simulink model "Simplified_Wind_Turbine_model"  (R2023b)
settings: Solver=ode23t  StartTime=0.0  StopTime=simT  RelTol=1e-3  AbsTol=1e-3
PreLoadFcn:
  | sscv_wind_turbine_input
values from neighbouring files (symbols this model uses):
  actuatorRampRate = 20    [sscv_wind_turbine_input.m]
  brakePressure = 100    [sscv_wind_turbine_input.m]
  controllerTimeConstant = 2    [sscv_wind_turbine_input.m]
  cumulativeStressThreshold = 1.5e6    (= 1500000)    [sscv_wind_turbine_input.m]
  generatorEfficiency = 90    [sscv_wind_turbine_input.m]
  iGenerationGain = 1    [sscv_wind_turbine_input.m]
  initialOperationTime = 0    [sscv_wind_turbine_input.m]
  inizialStressThreshold = 500e3    (= 500000)    [sscv_wind_turbine_input.m]
  maxPitchAngle = max(pitch)    [sscv_wind_turbine_input.m]
  minPitchAngle = min(pitch)    [sscv_wind_turbine_input.m]
  pGenerationGain = 0.1    [sscv_wind_turbine_input.m]
  pGeneratorBrakeLimit = 0.50    (= 0.5)    [sscv_wind_turbine_input.m]
  pitchBrakeAngle = 95    [sscv_wind_turbine_input.m]
  stressRateRelease = 0.05    [sscv_wind_turbine_input.m]
  transformerRatedPower = 1.8    [sscv_wind_turbine_input.m]
  turbineRatedPower = 1.5    [sscv_wind_turbine_input.m]
  vWindRated = 12    [sscv_wind_turbine_input.m]
  wAtGeneratorRatedPower = wTurbineCutOut*gearRatio    (= 1227.93)    [sscv_wind_turbine_input.m]
  wearRate = 0.033    [sscv_wind_turbine_input.m]
  wGeneratorBrakeLimit = 0.50    (= 0.5)    [sscv_wind_turbine_input.m]
  wTurbineCutOut = 22    [sscv_wind_turbine_input.m]
undefined symbols (not defined in the file or in its folder): Derating, mpptOmega, mpptPower, mpptWindSpeed
libraries: fl_lib x22, simulink x14, nesl_utility x11, sdl_lib x10, dspnetwork x3, simulink_extras x3
(part 1 of 2)
CloseFcn:
  | try,close(h_sscv_wind_turbine),end
  | clear h_sscv_wind_turbine
  | 
  | clear airDensity cp pitch TSR turbineRadius
  | clear vWindThreshold wThreshold vWindCutInLower
  | clear vWindCutOut vWindCutInUpper vWindRated
  | clear wTurbineCutIn wTurbineCutOut wTurbinePark
  | clear pitchBrakeAngle minPitchAngle maxPitchAngle
  | clear actuatorRampRate controllerTimeConstant
  | clear turbineRatedPower pGenerationGain
  | clear brakePressure brakeTorqueRadius
  | clear brakePistonArea brakeStaticFrictionCoeff
  | clear brakeKineticFrictionCoeff brakeClutchVelocityTol
  | clear brakeThresholdPressure numFrictionSurfaces
  | clear rotorBladeInertia generatorInertia
  | clear carrierShaftInertia stepShaftInertia
  | clear ringSunTeethRatio firstStepTeethRatio
  | clear secondStepTeethRatio windProfile
  | clear Derating gearRatio
  | clear generatorEfficiency mpptOmega mpptPower
  | clear generatorLumpedInductance generatorLumpedResistance
  | clear gridFrequency iGenerationGain
  | clear mpptWindSpeed transformerPrimaryVoltage
  | clear transformerRatedPower transformerSecondaryVoltage
  | clear wGeneratorBrakeLimit wAtGeneratorRatedPower
  | clear cpBraking simT pGeneratorBrakeLimit
  | clear windProfile1 windProfile2 windProfile3
  | clear numTSR
  | clear logsout_sscv_wind_turbine
  | clear simlog_sscv_wind_turbine
Description:
  | Wind Turbine
settings Model: SimulationMode=accelerator  Creator=The MathWorks, Inc.  LastModifiedBy=stefa
settings SolverCC: AutoScaleAbsTol=off  MaxConsecutiveMinStep=5  AlgebraicLoopSolver=TrustRegion  MaxZcPerStep=1
settings DataIOCC: SaveOutput=off  DSMLogging=off  SaveTime=off  ReturnWorkspaceOutputs=off  SignalLoggingName=logsout_sscv_wind_turbine
settings OptimizationCC: ReuseModelBlockBuffer=off
settings DebuggingCC: ReadBeforeWriteMsg=DisableAll  WriteAfterWriteMsg=DisableAll  WriteAfterReadMsg=DisableAll  MultiTaskDSMMsg=none  UnconnectedInputMsg=warning  UnconnectedOutputMsg=warning  UnconnectedLineMsg=warning
settings ModelReferenceCC: EnableRefExpFcnMdlSchedulingChecks=on
settings RTWCC: DLArmComputeVersion=19.05
settings SimscapeCC: SimscapeLogType=all  SimscapeLogSimulationStatistics=on  SimscapeLogName=simlog_sscv_wind_turbine  SimscapeLogDataHistory=10000000

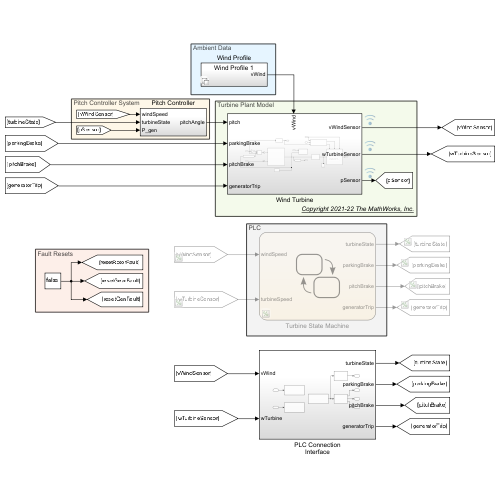
[thumbnail: Simulink's stored preview of the top-level diagram]
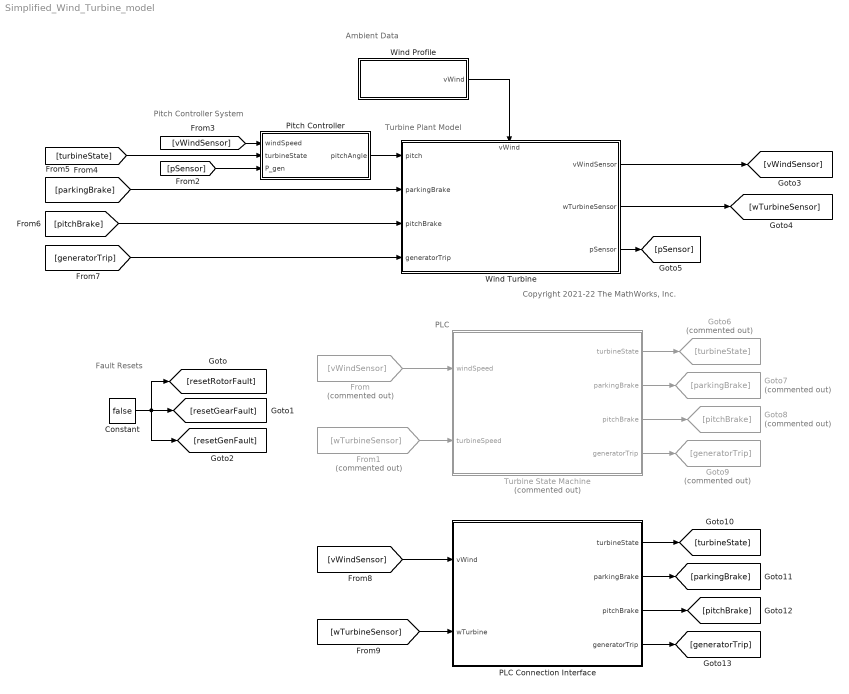
== system Simplified_Wind_Turbine_model ==
  note: Pitch Controller System
  note: Ambient Data
  note: Turbine Plant Model
  note: PLC
  note: Fault Resets
  note: Copyright 2021-22 The MathWorks, Inc.
  Constant : Constant  Value=false
  From : From  Commented=on  GotoTag=vWindSensor
  From1 : From  Commented=on  GotoTag=wTurbineSensor
  Goto6 : Goto  Commented=on  GotoTag=turbineState
  Goto7 : Goto  Commented=on  GotoTag=parkingBrake
  Goto8 : Goto  Commented=on  GotoTag=pitchBrake
  Goto9 : Goto  Commented=on  GotoTag=generatorTrip
  PLC Connection Interface : Subsystem
  Pitch Controller : Subsystem
  Turbine State Machine : Stateflow chart  Commented=on  TreatAsAtomicUnit=on
      settings: PortSchema="{\"entries\":[{\"content\":{\"sides\":[{\"content\":{\"connectorIds\":[\"In1\",\"In2\"]},\"type\":\"ConnectorPlacement.EquallySpacedRectSide\",\"uuid\":\"327e6e10-1b21-4a96-a275-8de2d485008c\"},{\"content\":{\"connectorIds\":[\"Out4\",\"Out2\",\"Out1\",\"Out3\"],\"side\":\"RIGHT\"},\"type\":\"ConnectorPlacement.EquallySpacedRectSide\",\"uuid\":\"1988adc6-59d9-4b8c-bf9e-88a31d7027f5\"},{\"content\":{\"side\":\"TOP\"},\"type\":\"ConnectorPlacement.EquallySpacedRectSide\",\"uuid\":\"79d1a7b7-1285-45ed-a7b5-26a06b144177\"}]},\"type\":\"ConnectorPlacement.EquallySpacedConnector\",\"uuid\":\"dd4ce8a9-3f97-44e2-8b7f-090ddfd1b400\"}],\"packageUris\":[\"http://schema.mathworks.com/mf0/Connector/R2020b\"],\"version\":\"1.0\"}"
  Wind Profile : Subsystem  Variant=on  VariantControl=Choice
  Wind Turbine : Subsystem
      settings: PortSchema="{\"entries\":[{\"content\":{\"sides\":[{\"content\":{\"connectorIds\":[\"In1\",\"In2\",\"In3\",\"In4\"]},\"type\":\"ConnectorPlacement.EquallySpacedRectSide\",\"uuid\":\"d7bfd4c3-1b44-42d5-b480-d0fc308ef744\"},{\"content\":{\"connectorIds\":[\"Out1\",\"Out2\",\"Out3\"],\"side\":\"RIGHT\"},\"type\":\"ConnectorPlacement.EquallySpacedRectSide\",\"uuid\":\"d62ac46e-8555-4545-8829-a8ccb57f6534\"},{\"content\":{\"connectorIds\":[\"In5\"],\"side\":\"TOP\"},\"type\":\"ConnectorPlacement.EquallySpacedRectSide\",\"uuid\":\"57f7c376-ec8e-430a-b1f8-8d8045a51355\"}]},\"type\":\"ConnectorPlacement.EquallySpacedConnector\",\"uuid\":\"f4d0f8a6-66a9-4a6a-8fc8-0ea319581c40\"}],\"packageUris\":[\"http://schema.mathworks.com/mf0/Connector/R2020b\"],\"version\":\"1.0\"}"
  wires:
  Pitch Controller/1(pitchAngle) -> Wind Turbine/1(pitch)
  Wind Profile/1(vWind) -> Wind Turbine/5(vWind)
  Constant/1 -> [resetGenFault], [resetRotorFault], [resetGearFault]
  Wind Turbine/1(vWindSensor) -> [vWindSensor]
  Wind Turbine/2(wTurbineSensor) -> [wTurbineSensor]
  Wind Turbine/3(pSensor) -> [pSensor]
  From/1 -> Turbine State Machine/1(windSpeed)
  From1/1 -> Turbine State Machine/2(turbineSpeed)
  [pSensor] -> Pitch Controller/3(P_gen)
  [vWindSensor] -> Pitch Controller/1(windSpeed)
  Turbine State Machine/4(turbineState) -> Goto6/1
  Turbine State Machine/2(parkingBrake) -> Goto7/1
  Turbine State Machine/1(pitchBrake) -> Goto8/1
  Turbine State Machine/3(generatorTrip) -> Goto9/1
  [turbineState] -> Pitch Controller/2(turbineState)
  [parkingBrake] -> Wind Turbine/2(parkingBrake)
  [pitchBrake] -> Wind Turbine/3(pitchBrake)
  [generatorTrip] -> Wind Turbine/4(generatorTrip)
  [vWindSensor] -> PLC Connection Interface/1(vWind)
  [wTurbineSensor] -> PLC Connection Interface/2(wTurbine)
  PLC Connection Interface/2(parkingBrake) -> [parkingBrake]
  PLC Connection Interface/1(turbineState) -> [turbineState]
  PLC Connection Interface/3(pitchBrake) -> [pitchBrake]
  PLC Connection Interface/4(generatorTrip) -> [generatorTrip]

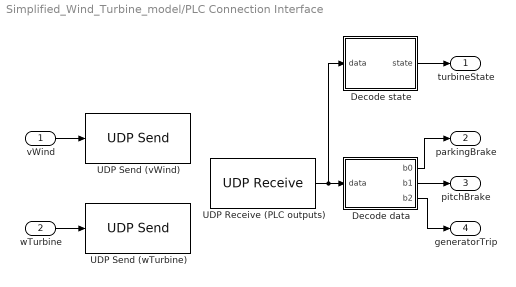
== system Simplified_Wind_Turbine_model/PLC Connection Interface ==
  vWind : Inport
  wTurbine : Inport  Port=2
  Decode data : MATLAB Function  TreatAsAtomicUnit=on
  Decode state : MATLAB Function  TreatAsAtomicUnit=on
  UDP Receive (PLC outputs) : dspnetwork/UDP Receive  localURL='0.0.0.0'  localPort=25000  remoteURL='0.0.0.0'  remotePort=-1  recvBufferSize=8192  dims=255  signalDatatype=uint8  isComplex=off  isVarSize=on  showBlockingTime=off  blockingTime=0  sampletime=0.1  blockPlatform=[]
      settings: LibrarySourceBlock=dspsrcs4/UDP Receive
  UDP Send (vWind) : dspnetwork/UDP Send  remoteURL='127.0.0.1'  remotePort=25000  localURL='0.0.0.0'  localPortSource=Automatically determine  localPort=-1  sendBufferSize=8192  sampletime=-1  blockPlatform=[]  separateLengthPort=0
      settings: LibrarySourceBlock=dspsnks4/UDP Send
  UDP Send (wTurbine) : dspnetwork/UDP Send  remoteURL='127.0.0.1'  remotePort=25000  localURL='0.0.0.0'  localPortSource=Automatically determine  localPort=-1  sendBufferSize=8192  sampletime=-1  blockPlatform=[]  separateLengthPort=0
      settings: LibrarySourceBlock=dspsnks4/UDP Send
  turbineState : Outport
  parkingBrake : Outport  Port=2
  pitchBrake : Outport  Port=3
  generatorTrip : Outport  Port=4
  wires:
  UDP Receive (PLC outputs)/1 -> Decode state/1(data), Decode data/1(data)
  Decode data/1(b0) -> parkingBrake/1
  Decode data/2(b1) -> pitchBrake/1
  Decode data/3(b2) -> generatorTrip/1
  Decode state/1(state) -> turbineState/1
  vWind/1 -> UDP Send (vWind)/1
  wTurbine/1 -> UDP Send (wTurbine)/1

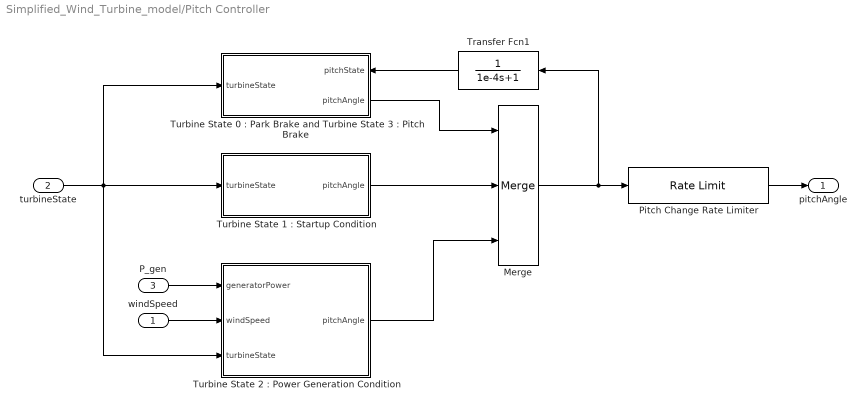
== system Simplified_Wind_Turbine_model/Pitch Controller ==
  windSpeed : Inport
  turbineState : Inport  Port=2
  P_gen : Inport  Port=3
  Merge : Merge  Inputs=3
  Pitch Change Rate Limiter : RateLimiter  RisingSlewLimit=actuatorRampRate  FallingSlewLimit=-actuatorRampRate  SampleTimeMode=inherited
  Transfer Fcn1 : TransferFcn  Denominator=[1e-4 1]
  "Turbine State 0 : Park Brake and Turbine State 3 : Pitch Brake" : Subsystem
      settings: PortSchema="{\"entries\":[{\"content\":{\"sides\":[{\"content\":{\"connectorIds\":[\"In1\"]},\"type\":\"ConnectorPlacement.EquallySpacedRectSide\",\"uuid\":\"c81c0fc4-0b31-4a43-acf3-ef02f67f12ef\"},{\"content\":{\"connectorIds\":[\"In2\",\"Out1\"],\"side\":\"RIGHT\"},\"type\":\"ConnectorPlacement.EquallySpacedRectSide\",\"uuid\":\"c20c9bc8-a4c7-4c6f-a8fa-fe8ff88298f7\"},{\"content\":{\"connectorIds\":[],\"side\":\"TOP\"},\"type\":\"ConnectorPlacement.EquallySpacedRectSide\",\"uuid\":\"2b845051-401f-423c-a453-0a1243a015d1\"}]},\"type\":\"ConnectorPlacement.EquallySpacedConnector\",\"uuid\":\"502647d6-ee95-4637-92b5-6d3c38784edf\"}],\"packageUris\":[\"http://schema.mathworks.com/mf0/Connector/R2020b\"],\"version\":\"1.0\"}"
  "Turbine State 1 : Startup Condition" : Subsystem
  "Turbine State 2 : Power Generation Condition" : Subsystem
  pitchAngle : Outport
  wires:
  Pitch Change Rate Limiter/1 -> pitchAngle/1
  turbineState/1 -> "Turbine State 2 : Power Generation Condition"/3(turbineState), "Turbine State 0 : Park Brake and Turbine State 3 : Pitch Brake"/1(turbineState), "Turbine State 1 : Startup Condition"/1(turbineState)
  P_gen/1 -> "Turbine State 2 : Power Generation Condition"/1(generatorPower)
  Merge/1 -> Pitch Change Rate Limiter/1, Transfer Fcn1/1
  "Turbine State 0 : Park Brake and Turbine State 3 : Pitch Brake"/1(pitchAngle) -> Merge/1
  "Turbine State 1 : Startup Condition"/1(pitchAngle) -> Merge/2
  "Turbine State 2 : Power Generation Condition"/1(pitchAngle) -> Merge/3
  windSpeed/1 -> "Turbine State 2 : Power Generation Condition"/2(windSpeed)
  Transfer Fcn1/1 -> "Turbine State 0 : Park Brake and Turbine State 3 : Pitch Brake"/2(pitchState)

== system Simplified_Wind_Turbine_model/Wind Profile ==
  Wind Profile 1 : Subsystem  VariantControl=windProfile1
  Wind Profile 2 : Subsystem  VariantControl=windProfile2
  Wind Profile 3 : Subsystem  VariantControl=windProfile3
  vWind : Outport

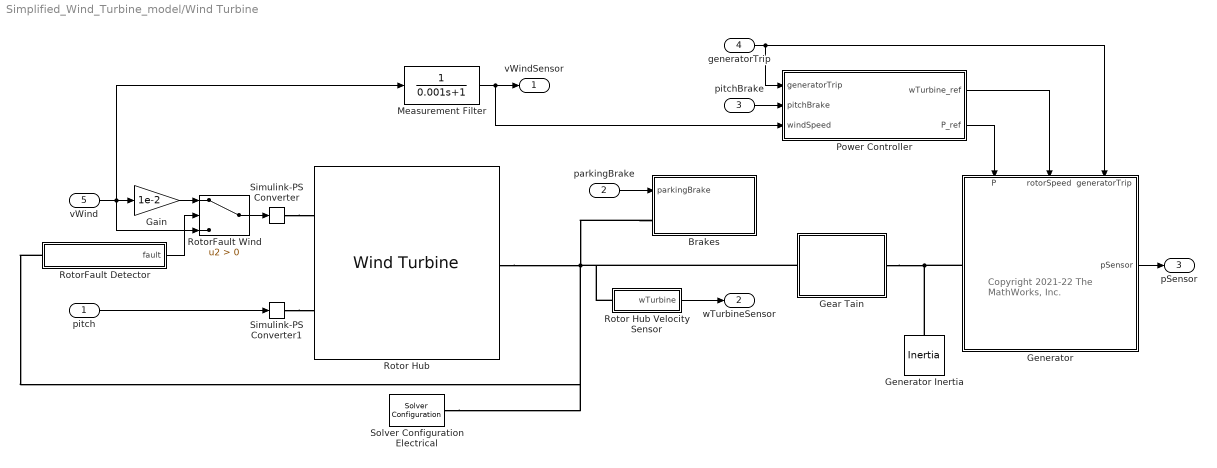
== system Simplified_Wind_Turbine_model/Wind Turbine ==
  note: Copyright 2021-22
      | The MathWorks, Inc.
  pitch : Inport
  parkingBrake : Inport  Port=2
  pitchBrake : Inport  Port=3
  generatorTrip : Inport  Port=4
  vWind : Inport  Port=5
  Brakes : Subsystem
  Gain : Gain  Gain=1e-2
  Gear Tain : Subsystem
  Generator : Subsystem
      settings: PortSchema="{\"entries\":[{\"content\":{\"sides\":[{\"content\":{\"connectorIds\":[\"LConn1\"]},\"type\":\"ConnectorPlacement.EquallySpacedRectSide\",\"uuid\":\"7b4c28dc-15ef-4b85-b689-03d2480b533c\"},{\"content\":{\"connectorIds\":[\"Out1\"],\"side\":\"RIGHT\"},\"type\":\"ConnectorPlacement.EquallySpacedRectSide\",\"uuid\":\"eb8f45a7-b1c6-4508-84d0-11c24daa06af\"},{\"content\":{\"connectorIds\":[\"In1\",\"In2\",\"In3\"],\"side\":\"TOP\"},\"type\":\"ConnectorPlacement.EquallySpacedRectSide\",\"uuid\":\"25f559ac-6538-4a67-925f-810721e5a71b\"},{\"content\":{\"side\":\"BOTTOM\"},\"type\":\"ConnectorPlacement.EquallySpacedRectSide\",\"uuid\":\"5619365a-5656-4cf0-a126-06e5a3f6ebac\"}]},\"type\":\"ConnectorPlacement.EquallySpacedConnector\",\"uuid\":\"4c1773ae-12cd-4fd2-b48a-ee13558bc69b\"}],\"packageUris\":[\"http://schema.mathworks.com/mf0/Connector/R2020b\"],\"version\":\"1.0\"}"
  Generator Inertia : fl_lib/Mechanical/Rotational Elements/Inertia  inertia=generatorInertia kg*m^2  num_ports=foundation.enum.numPorts2.one  w_specify=on  w_priority=None  w=0 rad/s  w_nominal_specify=off  w_nominal_unit=rad/s  w_nominal_value=1  t_specify=off  t_priority=None  t=0 N*m  t_nominal_specify=off  t_nominal_unit=N*m  t_nominal_value=1
  Measurement Filter : TransferFcn  Denominator=[0.001 1]
  Power Controller : Subsystem
  Rotor Hub : sdl_lib/Engines & Motors/Wind Turbine  model_thrust=false  R_rotor=turbineRadius m  pitch_TLU=pitch deg  lambda_TLU=TSR  Cp_TLU=cp  Ct_TLU=[0.0777, 0.1421, 0.3753, 0.6599, 0.8160, 0.9112, 0.9925, 1.0708, 1.1147; 0.0762, 0.1377, 0.3570, 0.5529, 0.6291, 0.6573, 0.6706, 0.6421, 0.6284; 0.0682, 0.1292, 0.3362, 0.4664, 0.4874, 0.4547, 0.3915, 0.2865, 0.2249; -0.05 * ones(1, 9)]  rho_air=airDensity kg/m^3  model_inertia=sdl.enum.model_inertia.on  rotor_inertia=rotorBladeInertia kg*m^2  init_rot_vel=0 rad/s  v_thr=0.01 m/s  w_thr=0.01 rad/s  expose_port_C=0
      settings: InternalSimscapePortConfiguration="{\"Bottom\":[],\"Left\":[{\"id\":\"vWind\",\"label\":\"V\",\"type\":\"input\"},{\"id\":\"pitch\",\"label\":\"β\",\"type\":\"input\"}],\"Right\":[{\"id\":\"R\",\"label\":\"R\",\"type\":\"foundation.mechanical.rotational.rotational\"}],\"Top\":[]}"
  Rotor Hub Velocity Sensor : Subsystem
  RotorFault Detector : Subsystem
  RotorFault Wind : Switch  Criteria=u2 > Threshold  SaturateOnIntegerOverflow=off  InputSameDT=off
  Simulink-PS Converter : nesl_utility/Simulink-PS Converter  PhysicalDomain=network_engine_domain  SubClassName=ps_input  LeftPortType=input  RightPortType=output  PseudoPeriodic=off  Frequencies=[]  NoiseDistribution=none  NoiseParameters=[]  Unit=m/s  AffineConversion=off  FilteringAndDerivatives=filter  SimscapeFilterOrder=1  InputFilterTimeConstant=0.001  UdotUserProvided=0
  Simulink-PS Converter1 : nesl_utility/Simulink-PS Converter  PhysicalDomain=network_engine_domain  SubClassName=ps_input  LeftPortType=input  RightPortType=output  PseudoPeriodic=off  Frequencies=[]  NoiseDistribution=none  NoiseParameters=[]  Unit=deg  AffineConversion=off  FilteringAndDerivatives=filter  SimscapeFilterOrder=1  InputFilterTimeConstant=0.001  UdotUserProvided=0
  Solver Configuration Electrical : nesl_utility/Solver Configuration  PhysicalDomain=network_engine_domain  SubClassName=solver  LeftPortType=input  RightPortType=generic  Tones=[]  Harmonics=[]  SimulateNoise=off  Profile=off  UseLocalSampling=off  EnableSwitchedLinearOptims=on  FrequencyDomain=off  UseCCode=off  RelTol=0.001  AbsTol=0.001  MinStep=1e-09  ToWorkspace=off  RevertToSquareIcSolve=off  NumHomotopyIterations=100  PhasorMode=off  PhasorModeNumHarmonics=1  ConsistencySolver=NEWTON_FTOL  IndexReductionMethod=DerivativeReplacement  DoDC=off  ResidualTolerance=1e-09  ConsistencyTolSource=GLOBAL  ConsistencyAbsTol=0.001  ConsistencyRelTol=0.001  ConsistencyTolFactor=0.001  UseLocalSolver=off  LocalSolverChoice=NE_TRAPEZOIDAL_ADVANCER  ResolveIndetEquations=on  FunctionEvalNumThread=1  LocalSolverSampleTime=1e-5  DoFixedCost=off  MaxNonlinIter=3  MaxModeIter=2  ComputeImpulses=off  ImpulseIterations=2  LinearAlgebra=auto  LinearAlgebraNumThread=0  EquationFormulation=NE_TIME_EF  DelaysMemoryBudget=1024  AutomaticFiltering=on  FilteringTimeConstant=0.001  PartitionStorageMethod=AS_NEEDED  PartitionMemoryBudget=1024  PartitionMethod=ROBUST  MultibodyUseLocalSolver=off  MultibodyLocalSolverChoice=ODE1  MultibodyLocalSolverSampleTime=0.001
  vWindSensor : Outport
  wTurbineSensor : Outport  Port=2
  pSensor : Outport  Port=3
  wires:
  Rotor Hub Velocity Sensor/1(wTurbine) -> wTurbineSensor/1
  Power Controller/2(P_ref) -> Generator/1(P)
  Generator/1(pSensor) -> pSensor/1
  parkingBrake/1 -> Brakes/1(parkingBrake)
  generatorTrip/1 -> Power Controller/1(generatorTrip), Generator/3(generatorTrip)
  Measurement Filter/1 -> vWindSensor/1, Power Controller/3(windSpeed)
  Power Controller/1(wTurbine_ref) -> Generator/2(rotorSpeed)
  pitchBrake/1 -> Power Controller/2(pitchBrake)
  pitch/1 -> Simulink-PS Converter1/1
  vWind/1 -> Measurement Filter/1, RotorFault Wind/3, Gain/1
  RotorFault Wind/1 -> Simulink-PS Converter/1
  RotorFault Detector/1(fault) -> RotorFault Wind/2
  Gain/1 -> RotorFault Wind/1
  connections:
  Generator/LConn1 -- Gear Tain/RConn1 -- Generator Inertia/LConn1
  Rotor Hub/RConn1 -- Solver Configuration Electrical/RConn1 -- RotorFault Detector/LConn1 -- Rotor Hub Velocity Sensor/LConn1 -- Gear Tain/LConn1 -- Brakes/LConn1
  Simulink-PS Converter/RConn1 -- Rotor Hub/LConn1
  Simulink-PS Converter1/RConn1 -- Rotor Hub/LConn2

== system Simplified_Wind_Turbine_model/Pitch Controller/Turbine State 0 : Park Brake and Turbine State 3 : Pitch Brake ==
  turbineState : Inport
  pitchState : Inport  Port=2
  Compare To Constant : simulink/Logic and Bit Operations/Compare To Constant  relop===  const=0  OutDataTypeStr=boolean
  Compare To Constant1 : simulink/Logic and Bit Operations/Compare To Constant  relop===  const=3  OutDataTypeStr=boolean
  OR : Logic  Operator=OR  IconShape=distinctive  AllPortsSameDT=off  OutDataTypeStr=boolean
  Turbine State 0 an 3 : Subsystem
  pitchAngle : Outport
  wires:
  Turbine State 0 an 3/1(pitchAngle) -> pitchAngle/1
  turbineState/1 -> Compare To Constant1/1, Compare To Constant/1
  pitchState/1 -> Turbine State 0 an 3/1(pitchState)
  OR/1 -> Turbine State 0 an 3/Enable
  Compare To Constant/1 -> OR/1
  Compare To Constant1/1 -> OR/2

== system Simplified_Wind_Turbine_model/Pitch Controller/Turbine State 1 : Startup Condition ==
  turbineState : Inport
  Compare To Constant : simulink/Logic and Bit Operations/Compare To Constant  relop===  const=1  OutDataTypeStr=boolean
  Turbine State 1 : Subsystem
  pitchAngle : Outport
  wires:
  turbineState/1 -> Compare To Constant/1
  Compare To Constant/1 -> Turbine State 1/Enable
  Turbine State 1/1(pitchAngle) -> pitchAngle/1

== system Simplified_Wind_Turbine_model/Pitch Controller/Turbine State 2 : Power Generation Condition ==
  generatorPower : Inport
  windSpeed : Inport  Port=2
  turbineState : Inport  Port=3
  Compare To Constant : simulink/Logic and Bit Operations/Compare To Constant  relop===  const=2  OutDataTypeStr=boolean
  Turbine State 2 : Subsystem
  pitchAngle : Outport
  wires:
  Turbine State 2/1(pitchAngle) -> pitchAngle/1
  Compare To Constant/1 -> Turbine State 2/Enable
  turbineState/1 -> Compare To Constant/1
  generatorPower/1 -> Turbine State 2/1(generatorPower)
  windSpeed/1 -> Turbine State 2/2(windSpeed)

== system Simplified_Wind_Turbine_model/Wind Profile/Wind Profile 1 ==
  Ramp : simulink/Sources/Ramp  slope=1  start=45  InitialOutput=15
  Saturation : Saturate  UpperLimit=22  LowerLimit=0
  vWind : Outport
  wires:
  Ramp/1 -> Saturation/1
  Saturation/1 -> vWind/1

== system Simplified_Wind_Turbine_model/Wind Profile/Wind Profile 2 ==
  Add : Sum  Inputs=+
  Mux : Mux  Inputs=3
  Ramp : simulink/Sources/Ramp  slope=0.7  start=0  InitialOutput=0
  Ramp1 : simulink/Sources/Ramp  slope=0.7  start=115  InitialOutput=0
  Ramp2 : simulink/Sources/Ramp  slope=-0.7  start=160  InitialOutput=0
  Saturation : Saturate  UpperLimit=10  LowerLimit=0
  Saturation1 : Saturate  UpperLimit=12  LowerLimit=0
  Saturation2 : Saturate  UpperLimit=0  LowerLimit=-7
  vWind : Outport
  wires:
  Saturation1/1 -> Mux/2
  Ramp/1 -> Saturation/1
  Ramp2/1 -> Saturation2/1
  Add/1 -> vWind/1
  Saturation/1 -> Mux/1
  Ramp1/1 -> Saturation1/1
  Mux/1 -> Add/1
  Saturation2/1 -> Mux/3

== system Simplified_Wind_Turbine_model/Wind Profile/Wind Profile 3 ==
  Ramp : simulink/Sources/Ramp  slope=1  start=45  InitialOutput=15
  Saturation : Saturate  UpperLimit=17  LowerLimit=0
  vWind : Outport
  wires:
  Ramp/1 -> Saturation/1
  Saturation/1 -> vWind/1

== system Simplified_Wind_Turbine_model/Wind Turbine/Brakes ==
  parkingBrake : Inport
  Disk Friction Clutch : sdl_lib/Clutches/Disc Friction Clutch  geometry_model=1  r_eff=brakeTorqueRadius m  d_o=150 mm  d_i=100 mm  nS=numFrictionSurfaces  piston_area=brakePistonArea m^2  unidirectional=0  friction_model=1  mu_w_vector=[1 1e8] rad/s  temperature_TLU=[280.0, 300.0, 320.0] K  mu_static=brakeStaticFrictionCoeff  mu_static_vector=[0.4, 0.38, 0.36]  mu_coulomb=brakeKineticFrictionCoeff  mu_coulomb_vector=[0.3 0.001]  mu_coulomb_temp_vector=[0.3, 0.28, 0.25]  mu_coulomb_matrix=[0.34, 0.32, 0.3; 0.3, 0.28, 0.25; 0.25, 0.2, 0.15]  mu_interp_method=1  mu_extrap_method=1  d_f=1  w_tol=brakeClutchVelocityTol rad/s  pressure_min=brakeThresholdPressure Pa  mu_visc=0 N*m/(rad/s)  initial_state_locked=sdl.enum.initial_lock.unlocked  enable_faults=simscape.enum.onoff.off  fault_type=sdl.enum.clutchFault.lock  external_fault=simscape.enum.onoff.off  temporal_fault=simscape.enum.onoff.off  fault_time=5 s  report_fault=simscape.enum.assert.action.none  thermal_mass=25 kJ/K  T_init=300 K
      settings: InternalSimscapePortConfiguration="{\"Bottom\":[],\"Left\":[{\"id\":\"P\",\"label\":\"P\",\"type\":\"input\"},{\"id\":\"B\",\"label\":\"B\",\"type\":\"foundation.mechanical.rotational.rotational\"}],\"Right\":[{\"id\":\"F\",\"label\":\"F\",\"type\":\"foundation.mechanical.rotational.rotational\"}],\"Top\":[]}"
  Engagement Pressure : Gain  Gain=brakePressure
  Mechanical Rotational Reference : fl_lib/Mechanical/Rotational Elements/Mechanical Rotational Reference
  Simulink-PS Converter : nesl_utility/Simulink-PS Converter  PhysicalDomain=network_engine_domain  SubClassName=ps_input  LeftPortType=input  RightPortType=output  PseudoPeriodic=off  Frequencies=[]  NoiseDistribution=none  NoiseParameters=[]  Unit=bar  AffineConversion=off  FilteringAndDerivatives=zero  SimscapeFilterOrder=1  InputFilterTimeConstant=0.005  UdotUserProvided=0
  R : PMIOPort  Tag=PMCPort  Side=Left
  wires:
  Engagement Pressure/1 -> Simulink-PS Converter/1
  parkingBrake/1 -> Engagement Pressure/1
  connections:
  Disk Friction Clutch/RConn1 -- Mechanical Rotational Reference/LConn1
  R/RConn1 -- Disk Friction Clutch/LConn2
  Simulink-PS Converter/RConn1 -- Disk Friction Clutch/LConn1

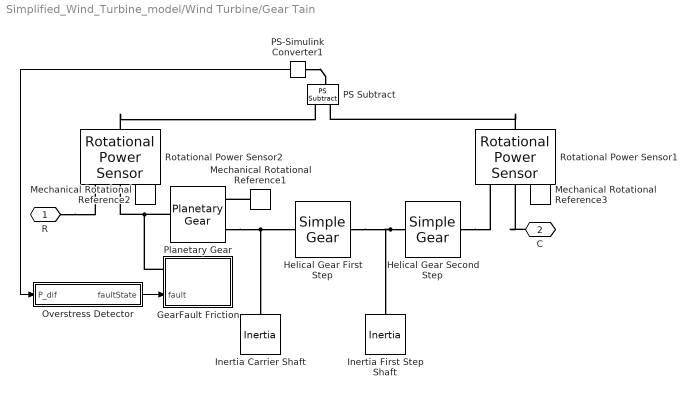
== system Simplified_Wind_Turbine_model/Wind Turbine/Gear Tain ==
  GearFault Friction : Subsystem
      settings: PortSchema="{\"entries\":[{\"content\":{\"sides\":[{\"content\":{\"connectorIds\":[\"LConn1\",\"In1\"]},\"type\":\"ConnectorPlacement.EquallySpacedRectSide\",\"uuid\":\"22e76782-3382-417d-ae5a-a7b1043ec7fc\"},{\"content\":{\"side\":\"RIGHT\"},\"type\":\"ConnectorPlacement.EquallySpacedRectSide\",\"uuid\":\"493f48a2-9880-444c-a7eb-314aeba6f102\"},{\"content\":{\"side\":\"TOP\"},\"type\":\"ConnectorPlacement.EquallySpacedRectSide\",\"uuid\":\"41df36c8-e029-4ee0-982b-378728ae749a\"}]},\"type\":\"ConnectorPlacement.EquallySpacedConnector\",\"uuid\":\"9c211b33-7010-4c0e-a899-cbcb07dff7a9\"}],\"packageUris\":[\"http://schema.mathworks.com/mf0/Connector/R2020b\"],\"version\":\"1.0\"}"
  Helical Gear First Step : sdl_lib/Gears/Simple Gear  ratio=firstStepTeethRatio  rotation_direction=sdl.enum.shaftOutputDirection.opposite  friction_model=sdl.enum.gear_efficiencies_load.constant  T_noload=0.1 N*m  T_nom=5 N*m  efficiency_nom=0.8  efficiency=0.95  temperature_TLU=[ 280 300 320 ] K  load_TLU=[ 1 5 10 ] N*m  efficiency_TLU=[ 0.95 0.9 0.85 ]  efficiency_TLU2=[ 0.85 0.8 0.75; 0.95 0.9 0.85; 0.85 0.8 0.7 ]  w_thr=0.01 rad/s  pwr_thr=0.001 W  enable_backlash=false  hardstop_model=simscape.enum.hardstop.smooth  backlash_distance=1e-3 mm  r_base=0.1 m  transition=1e-4 mm  backlash_stiffness=1e7 N/m  backlash_damping=1e6 N/(m/s)  coeff_rest=0  v_tol=0.001 m/s  f_tol=0 N  mu_visc=[ 0 0 ] N*m/(rad/s)  enable_faults=simscape.enum.onoff.off  efficiency_fault=0.05  external_fault=simscape.enum.onoff.off  temporal_fault=simscape.enum.onoff.off  fault_time=5 s  fault_angles=pi / 12 rad  report_fault=simscape.enum.assert.action.none  thermal_mass=50 J/K  temperature_specify=off  temperature_priority=High  temperature=300 K  temperature_nominal_specify=off  temperature_nominal_unit=K  temperature_nominal_value=1  x_backlash_specify=off  x_backlash_priority=None  x_backlash=0 mm  x_backlash_nominal_specify=off  x_backlash_nominal_unit=mm  x_backlash_nominal_value=1  f_hardstop_specify=off  f_hardstop_priority=None  f_hardstop=0 N  f_hardstop_nominal_specify=off  f_hardstop_nominal_unit=N  f_hardstop_nominal_value=1  v_backlash_specify=off  v_backlash_priority=None  v_backlash=0 m/s  v_backlash_nominal_specify=off  v_backlash_nominal_unit=m/s  v_backlash_nominal_value=1
  Helical Gear Second Step : sdl_lib/Gears/Simple Gear  ratio=secondStepTeethRatio  rotation_direction=sdl.enum.shaftOutputDirection.same  friction_model=sdl.enum.gear_efficiencies_load.constant  T_noload=0.1 N*m  T_nom=5 N*m  efficiency_nom=0.8  efficiency=0.95  temperature_TLU=[ 280 300 320 ] K  load_TLU=[ 1 5 10 ] N*m  efficiency_TLU=[ 0.95 0.9 0.85 ]  efficiency_TLU2=[ 0.85 0.8 0.75; 0.95 0.9 0.85; 0.85 0.8 0.7 ]  w_thr=0.01 rad/s  pwr_thr=0.001 W  enable_backlash=false  hardstop_model=simscape.enum.hardstop.smooth  backlash_distance=1e-3 mm  r_base=0.1 m  transition=1e-4 mm  backlash_stiffness=1e7 N/m  backlash_damping=1e6 N/(m/s)  coeff_rest=0  v_tol=0.001 m/s  f_tol=0 N  mu_visc=[ 0 0 ] N*m/(rad/s)  enable_faults=simscape.enum.onoff.off  efficiency_fault=0.05  external_fault=simscape.enum.onoff.off  temporal_fault=simscape.enum.onoff.off  fault_time=5 s  fault_angles=pi / 12 rad  report_fault=simscape.enum.assert.action.none  thermal_mass=50 J/K  temperature_specify=off  temperature_priority=High  temperature=300 K  temperature_nominal_specify=off  temperature_nominal_unit=K  temperature_nominal_value=1  x_backlash_specify=off  x_backlash_priority=None  x_backlash=0 mm  x_backlash_nominal_specify=off  x_backlash_nominal_unit=mm  x_backlash_nominal_value=1  f_hardstop_specify=off  f_hardstop_priority=None  f_hardstop=0 N  f_hardstop_nominal_specify=off  f_hardstop_nominal_unit=N  f_hardstop_nominal_value=1  v_backlash_specify=off  v_backlash_priority=None  v_backlash=0 m/s  v_backlash_nominal_specify=off  v_backlash_nominal_unit=m/s  v_backlash_nominal_value=1
  Inertia Carrier Shaft : fl_lib/Mechanical/Rotational Elements/Inertia  inertia=carrierShaftInertia kg*m^2  num_ports=foundation.enum.numPorts2.one  w_specify=on  w_priority=None  w=0 rad/s  w_nominal_specify=off  w_nominal_unit=rad/s  w_nominal_value=1  t_specify=off  t_priority=High  t=0 N*m  t_nominal_specify=off  t_nominal_unit=N*m  t_nominal_value=1
  Inertia First Step Shaft : fl_lib/Mechanical/Rotational Elements/Inertia  inertia=stepShaftInertia kg*m^2  num_ports=foundation.enum.numPorts2.one  w_specify=on  w_priority=None  w=0 rad/s  w_nominal_specify=off  w_nominal_unit=rad/s  w_nominal_value=1  t_specify=off  t_priority=High  t=0 N*m  t_nominal_specify=off  t_nominal_unit=N*m  t_nominal_value=1
  Mechanical Rotational Reference1 : fl_lib/Mechanical/Rotational Elements/Mechanical Rotational Reference
  Mechanical Rotational Reference2 : fl_lib/Mechanical/Rotational Elements/Mechanical Rotational Reference
  Mechanical Rotational Reference3 : fl_lib/Mechanical/Rotational Elements/Mechanical Rotational Reference
  Overstress Detector : Subsystem
  PS Subtract : fl_lib/Physical Signals/Functions/PS Subtract
  PS-Simulink Converter1 : nesl_utility/PS-Simulink Converter  PhysicalDomain=network_engine_domain  SubClassName=ps_output  LeftPortType=input  RightPortType=output  PseudoPeriodic=off  Frequencies=[]  VectorFormat=inherit  Unit=inherit  AffineConversion=off
  Planetary Gear : sdl_lib/Gears/Planetary Gear  rs_ratio=ringSunTeethRatio  friction_model=sdl.enum.gear_friction.constant  efficiency=[ 0.95 0.95 ]  temperature_TLU=[ 280 300 320 ] K  efficiency_sp_TLU=[ 0.95 0.9 0.85 ]  efficiency_rp_TLU=[ 0.95 0.9 0.85 ]  pwr_thr=[ 0.001 0.001 ] W  mu_visc=[0 0] N*m/(rad/s)  model_inertia=simscape.enum.onoff.off  planet_inertia=0.001 kg*m^2  thermal_mass=50 J/K  T_init=300 K
  Rotational Power Sensor1 : sdl_lib/Sensors/Rotational Power Sensor  measurement_type=sdl.enum.rotationalPowerSensorType.instantaneous  averaging_period=1 s  max_frequency=1000 Hz  max_speed=1000 rpm
      settings: InternalSimscapePortConfiguration="{\"Bottom\":[],\"Left\":[{\"id\":\"S\",\"label\":\"S\",\"type\":\"foundation.mechanical.rotational.rotational\"},{\"id\":\"R\",\"label\":\"R\",\"type\":\"foundation.mechanical.rotational.rotational\"},{\"id\":\"C\",\"label\":\"C\",\"type\":\"foundation.mechanical.rotational.rotational\"}],\"Right\":[{\"id\":\"P\",\"label\":\"P\",\"type\":\"output\"}],\"Top\":[]}"
  Rotational Power Sensor2 : sdl_lib/Sensors/Rotational Power Sensor  measurement_type=sdl.enum.rotationalPowerSensorType.instantaneous  averaging_period=1 s  max_frequency=1000 Hz  max_speed=1000 rpm
      settings: InternalSimscapePortConfiguration="{\"Bottom\":[],\"Left\":[{\"id\":\"S\",\"label\":\"S\",\"type\":\"foundation.mechanical.rotational.rotational\"},{\"id\":\"R\",\"label\":\"R\",\"type\":\"foundation.mechanical.rotational.rotational\"},{\"id\":\"C\",\"label\":\"C\",\"type\":\"foundation.mechanical.rotational.rotational\"}],\"Right\":[{\"id\":\"P\",\"label\":\"P\",\"type\":\"output\"}],\"Top\":[]}"
  R : PMIOPort  Side=Left
  C : PMIOPort  Port=2  Side=Right
  wires:
  Overstress Detector/1(faultState) -> GearFault Friction/1(fault)
  PS-Simulink Converter1/1 -> Overstress Detector/1(P_dif)
  connections:
  Planetary Gear/RConn2 -- Inertia Carrier Shaft/LConn1 -- Helical Gear First Step/RConn1
  Helical Gear Second Step/RConn1 -- Inertia First Step Shaft/LConn1 -- Helical Gear First Step/LConn1
  Mechanical Rotational Reference1/LConn1 -- Planetary Gear/RConn1
  Helical Gear Second Step/LConn1 -- Rotational Power Sensor1/LConn1
  C/RConn1 -- Rotational Power Sensor1/LConn2
  Mechanical Rotational Reference3/LConn1 -- Rotational Power Sensor1/LConn3
  Mechanical Rotational Reference2/LConn1 -- Rotational Power Sensor2/LConn3
  Planetary Gear/LConn1 -- GearFault Friction/LConn1 -- Rotational Power Sensor2/LConn2
  R/RConn1 -- Rotational Power Sensor2/LConn1
  Rotational Power Sensor1/RConn1 -- PS Subtract/LConn2
  PS-Simulink Converter1/LConn1 -- PS Subtract/RConn1
  Rotational Power Sensor2/RConn1 -- PS Subtract/LConn1

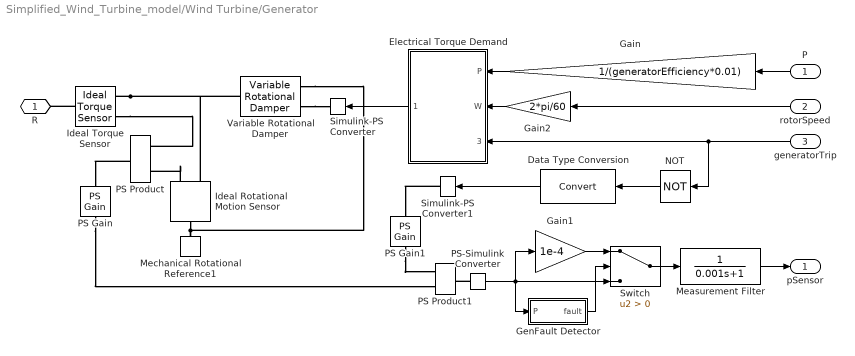
== system Simplified_Wind_Turbine_model/Wind Turbine/Generator ==
  P : Inport
  rotorSpeed : Inport  Port=2
  generatorTrip : Inport  Port=3
  Data Type Conversion : DataTypeConversion  SaturateOnIntegerOverflow=off  RndMeth=Floor
  Electrical Torque Demand : Subsystem
  Gain : Gain  Gain=1/(generatorEfficiency*0.01)
  Gain1 : Gain  Gain=1e-4
  Gain2 : Gain  Gain=2*pi/60
  GenFault Detector : Subsystem
  Ideal Rotational Motion Sensor : fl_lib/Mechanical/Mechanical Sensors/Ideal Rotational Motion Sensor  reference=foundation.enum.MeasurementReference.difference  acceleration_port=false  velocity_port=true  position_port=false  wrap_angle=simscape.enum.onoff.off  offset=0 rad
      settings: InternalSimscapePortConfiguration="{\"Bottom\":[],\"Left\":[{\"id\":\"R\",\"label\":\"R\",\"type\":\"foundation.mechanical.rotational.rotational\"}],\"Right\":[{\"id\":\"C\",\"label\":\"C\",\"type\":\"foundation.mechanical.rotational.rotational\"},{\"id\":\"W\",\"label\":\"W\",\"type\":\"output\"}],\"Top\":[]}"
  Ideal Torque Sensor : fl_lib/Mechanical/Mechanical Sensors/Ideal Torque Sensor
  Measurement Filter : TransferFcn  Denominator=[0.001 1]
  Mechanical Rotational Reference1 : fl_lib/Mechanical/Rotational Elements/Mechanical Rotational Reference
  NOT : Logic  Operator=NOT  IconShape=distinctive  AllPortsSameDT=off  OutDataTypeStr=boolean
  PS Gain : fl_lib/Physical Signals/Functions/PS Gain  gain=generatorEfficiency*0.01
  PS Gain1 : fl_lib/Physical Signals/Functions/PS Gain  gain=-1
  PS Product : fl_lib/Physical Signals/Functions/PS Product
  PS Product1 : fl_lib/Physical Signals/Functions/PS Product
  PS-Simulink Converter : nesl_utility/PS-Simulink Converter  PhysicalDomain=network_engine_domain  SubClassName=ps_output  LeftPortType=input  RightPortType=output  PseudoPeriodic=off  Frequencies=[]  VectorFormat=inherit  Unit=MW  AffineConversion=off
  Simulink-PS Converter : nesl_utility/Simulink-PS Converter  PhysicalDomain=network_engine_domain  SubClassName=ps_input  LeftPortType=input  RightPortType=output  PseudoPeriodic=off  Frequencies=[]  NoiseDistribution=none  NoiseParameters=[]  Unit=N*m/(rad/s)  AffineConversion=off  FilteringAndDerivatives=provide  SimscapeFilterOrder=1  InputFilterTimeConstant=0.001  UdotUserProvided=0
  Simulink-PS Converter1 : nesl_utility/Simulink-PS Converter  PhysicalDomain=network_engine_domain  SubClassName=ps_input  LeftPortType=input  RightPortType=output  PseudoPeriodic=off  Frequencies=[]  NoiseDistribution=none  NoiseParameters=[]  Unit=1  AffineConversion=off  FilteringAndDerivatives=provide  SimscapeFilterOrder=1  InputFilterTimeConstant=0.001  UdotUserProvided=0
  Switch : Switch  Criteria=u2 > Threshold  SaturateOnIntegerOverflow=off  InputSameDT=off
  Variable Rotational Damper : sdl_lib/Couplings & Drives/Springs & Dampers/Variable Rotational Damper  Bmin=1e-3 N*m*s/rad
      settings: InternalSimscapePortConfiguration="{\"Bottom\":[],\"Left\":[{\"id\":\"B\",\"label\":\"B\",\"type\":\"input\"},{\"id\":\"R\",\"label\":\"R\",\"type\":\"foundation.mechanical.rotational.rotational\"}],\"Right\":[{\"id\":\"C\",\"label\":\"C\",\"type\":\"foundation.mechanical.rotational.rotational\"}],\"Top\":[]}"
  R : PMIOPort  Side=Left
  pSensor : Outport
  wires:
  Gain/1 -> Electrical Torque Demand/1(P)
  Gain2/1 -> Electrical Torque Demand/2(W)
  generatorTrip/1 -> NOT/1, Electrical Torque Demand/3(generatorTrip)
  rotorSpeed/1 -> Gain2/1
  Electrical Torque Demand/1(Damping) -> Simulink-PS Converter/1
  P/1 -> Gain/1
  Measurement Filter/1 -> pSensor/1
  NOT/1 -> Data Type Conversion/1
  Data Type Conversion/1 -> Simulink-PS Converter1/1
  PS-Simulink Converter/1 -> GenFault Detector/1(P), Gain1/1, Switch/3
  Gain1/1 -> Switch/1
  Switch/1 -> Measurement Filter/1
  GenFault Detector/1(fault) -> Switch/2
  connections:
  Ideal Torque Sensor/RConn1 -- Variable Rotational Damper/RConn1 -- Ideal Rotational Motion Sensor/RConn1
  Ideal Torque Sensor/LConn1 -- R/RConn1
  Ideal Rotational Motion Sensor/RConn2 -- PS Product/LConn1
  Variable Rotational Damper/LConn1 -- Simulink-PS Converter/RConn1
  Ideal Torque Sensor/RConn2 -- PS Product/LConn2
  PS Product/RConn1 -- PS Gain/LConn1
  Ideal Rotational Motion Sensor/LConn1 -- Variable Rotational Damper/LConn2 -- Mechanical Rotational Reference1/LConn1
  PS Gain/RConn1 -- PS Product1/LConn2
  PS Gain1/RConn1 -- PS Product1/LConn1
  PS-Simulink Converter/LConn1 -- PS Product1/RConn1
  Simulink-PS Converter1/RConn1 -- PS Gain1/LConn1

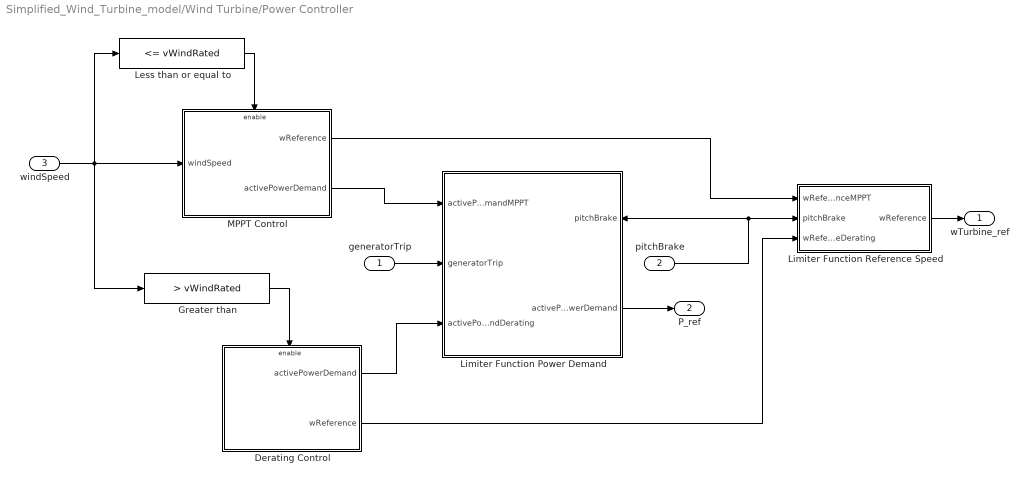
== system Simplified_Wind_Turbine_model/Wind Turbine/Power Controller ==
  generatorTrip : Inport
  pitchBrake : Inport  Port=2
  windSpeed : Inport  Port=3
  Derating Control : Subsystem
  Greater than : simulink/Logic and Bit Operations/Compare To Constant  relop=>  const=vWindRated  OutDataTypeStr=boolean
  Less than or equal to : simulink/Logic and Bit Operations/Compare To Constant  relop=<=  const=vWindRated  OutDataTypeStr=boolean
  Limiter Function Power Demand : Subsystem
      settings: PortSchema="{\"entries\":[{\"content\":{\"sides\":[{\"content\":{\"connectorIds\":[\"In1\",\"In2\",\"In3\"]},\"type\":\"ConnectorPlacement.EquallySpacedRectSide\",\"uuid\":\"b03cf57d-370b-4fa1-bd93-9b836e03697e\"},{\"content\":{\"connectorIds\":[\"In4\",\"Out1\"],\"side\":\"RIGHT\"},\"type\":\"ConnectorPlacement.EquallySpacedRectSide\",\"uuid\":\"152758c3-43df-447a-a50f-afca466b3eeb\"},{\"content\":{\"connectorIds\":[],\"side\":\"TOP\"},\"type\":\"ConnectorPlacement.EquallySpacedRectSide\",\"uuid\":\"d053be3f-8f1f-4fa1-8d53-3d41a1fdecc7\"}]},\"type\":\"ConnectorPlacement.EquallySpacedConnector\",\"uuid\":\"ad588a80-a06e-49b6-a4d2-a4be271ff49a\"}],\"packageUris\":[\"http://schema.mathworks.com/mf0/Connector/R2020b\"],\"version\":\"1.0\"}"
  Limiter Function Reference Speed : Subsystem
  MPPT Control : Subsystem
  wTurbine_ref : Outport
  P_ref : Outport  Port=2
  wires:
  windSpeed/1 -> Greater than/1, Less than or equal to/1, MPPT Control/1(windSpeed)
  Less than or equal to/1 -> MPPT Control/Enable
  Greater than/1 -> Derating Control/Enable
  MPPT Control/2(activePowerDemand) -> Limiter Function Power Demand/1(activePowerDemandMPPT)
  generatorTrip/1 -> Limiter Function Power Demand/2(generatorTrip)
  Derating Control/1(activePowerDemand) -> Limiter Function Power Demand/3(activePowerDemandDerating)
  Limiter Function Power Demand/1(activePowerDemand) -> P_ref/1
  pitchBrake/1 -> Limiter Function Reference Speed/2(pitchBrake), Limiter Function Power Demand/4(pitchBrake)
  MPPT Control/1(wReference) -> Limiter Function Reference Speed/1(wReferenceMPPT)
  Derating Control/2(wReference) -> Limiter Function Reference Speed/3(wReferenceDerating)
  Limiter Function Reference Speed/1(wReference) -> wTurbine_ref/1

== system Simplified_Wind_Turbine_model/Wind Turbine/Rotor Hub Velocity Sensor ==
  Ideal Rotational Motion Sensor : fl_lib/Mechanical/Mechanical Sensors/Ideal Rotational Motion Sensor  reference=foundation.enum.MeasurementReference.difference  acceleration_port=false  velocity_port=true  position_port=false  wrap_angle=simscape.enum.onoff.off  offset=0 rad
      settings: InternalSimscapePortConfiguration="{\"Bottom\":[],\"Left\":[{\"id\":\"R\",\"label\":\"R\",\"type\":\"foundation.mechanical.rotational.rotational\"}],\"Right\":[{\"id\":\"C\",\"label\":\"C\",\"type\":\"foundation.mechanical.rotational.rotational\"},{\"id\":\"W\",\"label\":\"W\",\"type\":\"output\"}],\"Top\":[]}"
  Measurement Filter : TransferFcn  Denominator=[0.001 1]
  Mechanical Rotational Reference2 : fl_lib/Mechanical/Rotational Elements/Mechanical Rotational Reference
  PS-Simulink Converter : nesl_utility/PS-Simulink Converter  PhysicalDomain=network_engine_domain  SubClassName=ps_output  LeftPortType=input  RightPortType=output  PseudoPeriodic=off  Frequencies=[]  VectorFormat=1-D array  Unit=rpm  AffineConversion=off
  R : PMIOPort  Side=Left
  wTurbine : Outport
  wires:
  PS-Simulink Converter/1 -> Measurement Filter/1
  Measurement Filter/1 -> wTurbine/1
  connections:
  Ideal Rotational Motion Sensor/RConn2 -- PS-Simulink Converter/LConn1
  Ideal Rotational Motion Sensor/LConn1 -- R/RConn1
  Ideal Rotational Motion Sensor/RConn1 -- Mechanical Rotational Reference2/LConn1

== system Simplified_Wind_Turbine_model/Wind Turbine/RotorFault Detector ==
  Compare To Constant : simulink/Logic and Bit Operations/Compare To Constant  relop=>  const=wTurbineCutOut*1.3  OutDataTypeStr=boolean
  Ideal Rotational Motion Sensor : fl_lib/Mechanical/Mechanical Sensors/Ideal Rotational Motion Sensor  reference=foundation.enum.MeasurementReference.difference  acceleration_port=false  velocity_port=true  position_port=false  wrap_angle=simscape.enum.onoff.off  offset=0 rad
      settings: InternalSimscapePortConfiguration="{\"Bottom\":[],\"Left\":[{\"id\":\"R\",\"label\":\"R\",\"type\":\"foundation.mechanical.rotational.rotational\"}],\"Right\":[{\"id\":\"C\",\"label\":\"C\",\"type\":\"foundation.mechanical.rotational.rotational\"},{\"id\":\"W\",\"label\":\"W\",\"type\":\"output\"}],\"Top\":[]}"
  Mechanical Rotational Reference : fl_lib/Mechanical/Rotational Elements/Mechanical Rotational Reference
  PS-Simulink Converter : nesl_utility/PS-Simulink Converter  PhysicalDomain=network_engine_domain  SubClassName=ps_output  LeftPortType=input  RightPortType=output  PseudoPeriodic=off  Frequencies=[]  VectorFormat=inherit  Unit=rpm  AffineConversion=off
  S-R Flip-Flop : simulink_extras/Flip Flops/S-R Flip-Flop  initial_condition=0
  Terminator : Terminator
  R : PMIOPort  Side=Left
  fault : Outport
  wires:
  PS-Simulink Converter/1 -> Compare To Constant/1
  Compare To Constant/1 -> S-R Flip-Flop/1
  S-R Flip-Flop/1 -> fault/1
  [resetRotorFault] -> S-R Flip-Flop/2
  S-R Flip-Flop/2 -> Terminator/1
  connections:
  Ideal Rotational Motion Sensor/RConn2 -- PS-Simulink Converter/LConn1
  Ideal Rotational Motion Sensor/LConn1 -- R/RConn1
  Ideal Rotational Motion Sensor/RConn1 -- Mechanical Rotational Reference/LConn1

== system Simplified_Wind_Turbine_model/Pitch Controller/Turbine State 0 : Park Brake and Turbine State 3 : Pitch Brake/Turbine State 0 an 3 ==
  note: Turbine State 0 & 3: Park & Pitch Brake
  pitchState : Inport
  Enable : EnablePort  StatesWhenEnabling=reset
  Constant : Constant  Value=pitchBrakeAngle
  Constant1 : Constant
  Controller : TransferFcn  Denominator="[controllerTimeConstant  1]"
  Integrator : Integrator
  Switch : Switch  Criteria=u2 > Threshold  Threshold=controllerTimeConstant*log(1-(maxPitchAngle/pitchBrakeAngle))*(-1.01)  SaturateOnIntegerOverflow=off  InputSameDT=off
  pitchAngle : Outport
  wires:
  Integrator/1 -> Switch/2
  pitchState/1 -> Switch/3
  Constant1/1 -> Integrator/1
  Constant/1 -> Controller/1
  Controller/1 -> Switch/1
  Switch/1 -> pitchAngle/1

== system Simplified_Wind_Turbine_model/Pitch Controller/Turbine State 1 : Startup Condition/Turbine State 1 ==
  note: Turbine State 1: Startup
  Enable : EnablePort  StatesWhenEnabling=reset
  Constant : Constant  Value=minPitchAngle
  Saturation : Saturate  UpperLimit=maxPitchAngle  LowerLimit=minPitchAngle
  Transfer Fcn : TransferFcn  Denominator=[controllerTimeConstant 1]
  pitchAngle : Outport
  wires:
  Constant/1 -> Transfer Fcn/1
  Saturation/1 -> pitchAngle/1
  Transfer Fcn/1 -> Saturation/1

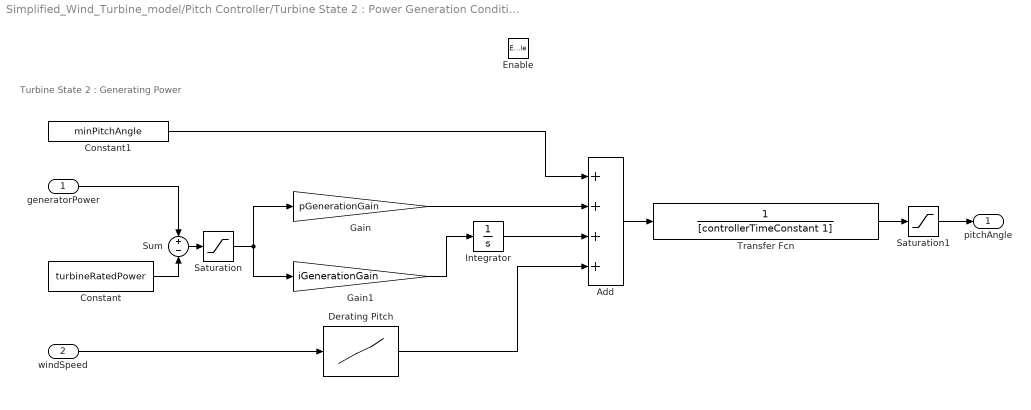
== system Simplified_Wind_Turbine_model/Pitch Controller/Turbine State 2 : Power Generation Condition/Turbine State 2 ==
  note: Turbine State 2 : Generating Power
  generatorPower : Inport
  windSpeed : Inport  Port=2
  Enable : EnablePort  StatesWhenEnabling=reset
  Add : Sum  Inputs=++++
  Constant : Constant  Value=turbineRatedPower
  Constant1 : Constant  Value=minPitchAngle
  Derating Pitch : Lookup_n-D  NumberOfTableDimensions=1  BreakpointsForDimension1=Derating(:,1)  BeginIndexSearchUsingPreviousIndexResult=on  Table=Derating(:,2)-minPitchAngle  InternalRulePriority=Speed  RndMeth=Simplest
  Gain : Gain  Gain=pGenerationGain
  Gain1 : Gain  Gain=iGenerationGain
  Integrator : Integrator
  Saturation : Saturate  UpperLimit=inf  LowerLimit=0
  Saturation1 : Saturate  UpperLimit=maxPitchAngle  LowerLimit=minPitchAngle
  Sum : Sum  Inputs=+-
  Transfer Fcn : TransferFcn  Denominator=[controllerTimeConstant 1]
  pitchAngle : Outport
  wires:
  Saturation1/1 -> pitchAngle/1
  Gain/1 -> Add/2
  Constant1/1 -> Add/1
  Add/1 -> Transfer Fcn/1
  generatorPower/1 -> Sum/1
  Constant/1 -> Sum/2
  Sum/1 -> Saturation/1
  Saturation/1 -> Gain/1, Gain1/1
  Transfer Fcn/1 -> Saturation1/1
  Integrator/1 -> Add/3
  Gain1/1 -> Integrator/1
  windSpeed/1 -> Derating Pitch/1
  Derating Pitch/1 -> Add/4

== system Simplified_Wind_Turbine_model/Wind Turbine/Gear Tain/GearFault Friction ==
  fault : Inport
  Data Type Conversion : DataTypeConversion  SaturateOnIntegerOverflow=off  RndMeth=Floor
  GearFault1 : sdl_lib/Clutches/Logic-Controlled Clutch  transition_model=sdl.enum.transitionModel.timeConstant  transition_time_constant=0.03 s  t_friction=1e+6 N*m  t_locked=1.5e+6 N*m  w_tol=0.001 rad/s  initial_state_locked=sdl.enum.initial_lock.unlocked
      settings: InternalSimscapePortConfiguration="{\"Bottom\":[],\"Left\":[{\"id\":\"E\",\"label\":\"E\",\"type\":\"input\"},{\"id\":\"B\",\"label\":\"B\",\"type\":\"foundation.mechanical.rotational.rotational\"}],\"Right\":[{\"id\":\"F\",\"label\":\"F\",\"type\":\"foundation.mechanical.rotational.rotational\"}],\"Top\":[]}"
  GearFault2 : sdl_lib/Clutches/Logic-Controlled Clutch  transition_model=sdl.enum.transitionModel.timeConstant  transition_time_constant=0.001 s  t_friction=0.5e+6 N*m  t_locked=1e+6 N*m  w_tol=0.001 rad/s  initial_state_locked=sdl.enum.initial_lock.unlocked
      settings: InternalSimscapePortConfiguration="{\"Bottom\":[],\"Left\":[{\"id\":\"E\",\"label\":\"E\",\"type\":\"input\"},{\"id\":\"B\",\"label\":\"B\",\"type\":\"foundation.mechanical.rotational.rotational\"}],\"Right\":[{\"id\":\"F\",\"label\":\"F\",\"type\":\"foundation.mechanical.rotational.rotational\"}],\"Top\":[]}"
  Ideal Rotational Motion Sensor : fl_lib/Mechanical/Mechanical Sensors/Ideal Rotational Motion Sensor  reference=foundation.enum.MeasurementReference.difference  acceleration_port=false  velocity_port=false  position_port=true  wrap_angle=true  offset=0 rad
      settings: InternalSimscapePortConfiguration="{\"Bottom\":[],\"Left\":[{\"id\":\"R\",\"label\":\"R\",\"type\":\"foundation.mechanical.rotational.rotational\"}],\"Right\":[{\"id\":\"C\",\"label\":\"C\",\"type\":\"foundation.mechanical.rotational.rotational\"},{\"id\":\"A\",\"label\":\"A\",\"type\":\"output\"}],\"Top\":[]}"
  Mechanical Rotational Reference2 : fl_lib/Mechanical/Rotational Elements/Mechanical Rotational Reference
  PS Product : fl_lib/Physical Signals/Functions/PS Product
  Simulink-PS Converter : nesl_utility/Simulink-PS Converter  PhysicalDomain=network_engine_domain  SubClassName=ps_input  LeftPortType=input  RightPortType=output  PseudoPeriodic=off  Frequencies=[]  NoiseDistribution=none  NoiseParameters=[]  Unit=1  AffineConversion=off  FilteringAndDerivatives=provide  SimscapeFilterOrder=1  InputFilterTimeConstant=0.001  UdotUserProvided=0
  R : PMIOPort  Side=Left
  wires:
  fault/1 -> Data Type Conversion/1
  Data Type Conversion/1 -> Simulink-PS Converter/1
  connections:
  GearFault1/RConn1 -- Mechanical Rotational Reference2/LConn1 -- Ideal Rotational Motion Sensor/RConn1 -- GearFault2/RConn1
  PS Product/RConn1 -- GearFault2/LConn1
  GearFault1/LConn1 -- PS Product/LConn2 -- Simulink-PS Converter/RConn1
  Ideal Rotational Motion Sensor/RConn2 -- PS Product/LConn1
  GearFault2/LConn2 -- GearFault1/LConn2 -- R/RConn1 -- Ideal Rotational Motion Sensor/LConn1

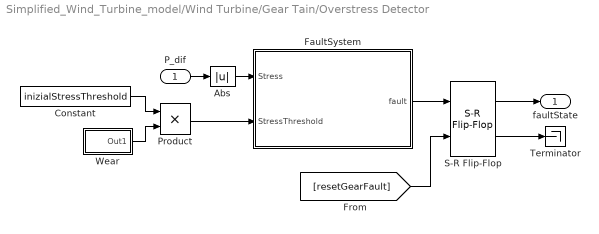
== system Simplified_Wind_Turbine_model/Wind Turbine/Gear Tain/Overstress Detector ==
  P_dif : Inport
  Abs : Abs  SaturateOnIntegerOverflow=off
  Constant : Constant  Value=inizialStressThreshold
  FaultSystem : Subsystem
  Product : Product
  S-R Flip-Flop : simulink_extras/Flip Flops/S-R Flip-Flop  initial_condition=0
  Terminator : Terminator
  Wear : Subsystem
  faultState : Outport
  wires:
  S-R Flip-Flop/1 -> faultState/1
  Abs/1 -> FaultSystem/1(Stress)
  FaultSystem/1(fault) -> S-R Flip-Flop/1
  P_dif/1 -> Abs/1
  Wear/1(Out1) -> Product/2
  Constant/1 -> Product/1
  Product/1 -> FaultSystem/2(StressThreshold)
  S-R Flip-Flop/2 -> Terminator/1
  [resetGearFault] -> S-R Flip-Flop/2

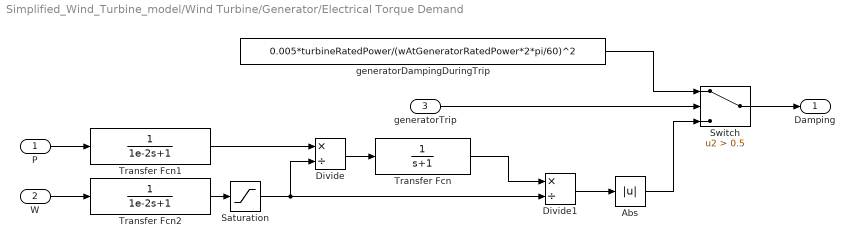
== system Simplified_Wind_Turbine_model/Wind Turbine/Generator/Electrical Torque Demand ==
  P : Inport
  W : Inport  Port=2
  generatorTrip : Inport  Port=3
  Abs : Abs  SaturateOnIntegerOverflow=off
  Divide : Product  Inputs=*/
  Divide1 : Product  Inputs=*/
  Saturation : Saturate  UpperLimit=inf  LowerLimit=0.2*wAtGeneratorRatedPower*2*pi/60
  Switch : Switch  Criteria=u2 > Threshold  Threshold=0.5  SaturateOnIntegerOverflow=off  InputSameDT=off
  Transfer Fcn : TransferFcn  Denominator=[1 1]
  Transfer Fcn1 : TransferFcn  Denominator=[1e-2 1]
  Transfer Fcn2 : TransferFcn  Denominator=[1e-2 1]
  generatorDampingDuringTrip : Constant  Value=0.005*turbineRatedPower/(wAtGeneratorRatedPower*2*pi/60)^2
  Damping : Outport
  wires:
  Divide1/1 -> Abs/1
  Divide/1 -> Transfer Fcn/1
  Transfer Fcn/1 -> Divide1/1
  W/1 -> Transfer Fcn2/1
  Transfer Fcn1/1 -> Divide/1
  P/1 -> Transfer Fcn1/1
  Transfer Fcn2/1 -> Saturation/1
  Saturation/1 -> Divide1/2, Divide/2
  generatorTrip/1 -> Switch/2
  Abs/1 -> Switch/3
  Switch/1 -> Damping/1
  generatorDampingDuringTrip/1 -> Switch/1

== system Simplified_Wind_Turbine_model/Wind Turbine/Generator/GenFault Detector ==
  P : Inport
  Compare To Constant : simulink/Logic and Bit Operations/Compare To Constant  relop=>  const=transformerRatedPower*1.35  OutDataTypeStr=boolean
  S-R Flip-Flop : simulink_extras/Flip Flops/S-R Flip-Flop  initial_condition=0
  Terminator : Terminator
  fault : Outport
  wires:
  P/1 -> Compare To Constant/1
  Compare To Constant/1 -> S-R Flip-Flop/1
  S-R Flip-Flop/1 -> fault/1
  S-R Flip-Flop/2 -> Terminator/1
  [resetGenFault] -> S-R Flip-Flop/2

== system Simplified_Wind_Turbine_model/Wind Turbine/Power Controller/Derating Control ==
  Enable : EnablePort  StatesWhenEnabling=reset
  Constant : Constant  Value=turbineRatedPower
  Constant1 : Constant  Value=wAtGeneratorRatedPower
  Gain : Gain  Gain=100/generatorEfficiency
  MW to W : Gain  Gain=1e6
  activePowerDemand : Outport
  wReference : Outport  Port=2
  wires:
  Constant1/1 -> wReference/1
  MW to W/1 -> activePowerDemand/1
  Constant/1 -> Gain/1
  Gain/1 -> MW to W/1
